simulink model "RobotX_SLAMdataCollect"  (R2014a)
settings: Solver=FixedStepDiscrete  StartTime=0.0  StopTime=inf  FixedStep=.25  RelTol=1e-3
undefined symbols (not defined in the file): Com1, Com2, Com3, Com4, DiscIntNeverNeededParam, standard
libraries: xpcseriallib x11, slrtlib x4, simulink x1, speedgoatlib x1, speedgoatlib_IO102 x1
settings Model: BufferReuse=off  Creator=wildcat  LastModifiedBy=wildcat
settings SolverCC: EnableConcurrentExecution=on
settings DataIOCC: SignalLoggingSaveFormat=ModelDataLogs
settings OptimizationCC: BlockReduction=off  OptimizeBlockIOStorage=off  BufferReuse=off  GlobalBufferReuse=off  ExpressionFolding=off  LocalBlockOutputs=off
settings DebuggingCC: UnderspecifiedInitializationDetection=Classic  StateNameClashWarn=warning
settings HardwareCC: ProdIntDivRoundTo=Zero  ProdEndianess=LittleEndian  ProdHWDeviceType=Generic->32-bit x86 compatible
settings RTWCC: SystemTargetFile=slrt.tlc  TemplateMakefile=slrt_default_tmf  Description=Simulink Real-Time  ProcessScript=slrt_make_rtw_hook  RTWCompilerOptimization=On
settings SimulinkRealTimeCC: GeneratePreprocessorConditionals=Disable all  EnableShiftOperators=on

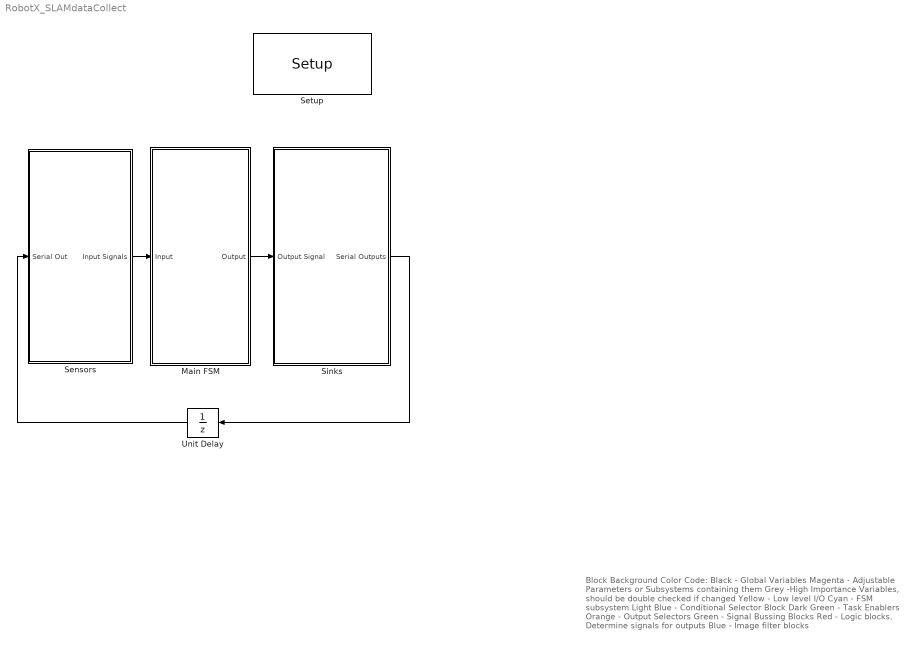
== system RobotX_SLAMdataCollect ==
  note: Block Background Color Code:
      | Black - Global Variables
      | Magenta - Adjustable Parameters or Subsystems containing them
      | Grey -High Importance Variables, should be double checked if changed
      | Yellow - Low level I/O
      | Cyan - FSM subsystem
      | Light Blue - Conditional Selector Block
      | Dark Green - Task Enablers
      | Orange - Output Selectors
      | Green - Signal Bussing Blocks
      | Red - Logic blocks. Determine signals for outputs
      | Blue - Image filter blocks
  Main FSM : Subsystem
  Sensors : Subsystem
  Setup : speedgoatlib_IO102/Setup  group=Digital output setup  id=1  range=+-5V  cal=off  pciSlot=-1  adChannelMode=Multiple-channel (enter number of channels below)  adChannel=16  adCoupling=Differential  daChannel=[1,2,3,4]  daReset=[1]  daInitValue=[0]  diChannel=[1,2,3,4,5,6,7,8]  doChannel=[1,2,3,4,5,6,7,8]  doReset=[1]  doInitValue=[0]
  Sinks : Subsystem
  Unit Delay : UnitDelay  SampleTime=-1
  wires:
  Main FSM/1(Output) -> Sinks/1(Output Signal)
  Sensors/1(Input Signals) -> Main FSM/1(Input)
  Sinks/1(Serial Outputs) -> Unit Delay/1
  Unit Delay/1 -> Sensors/1(Serial Out)

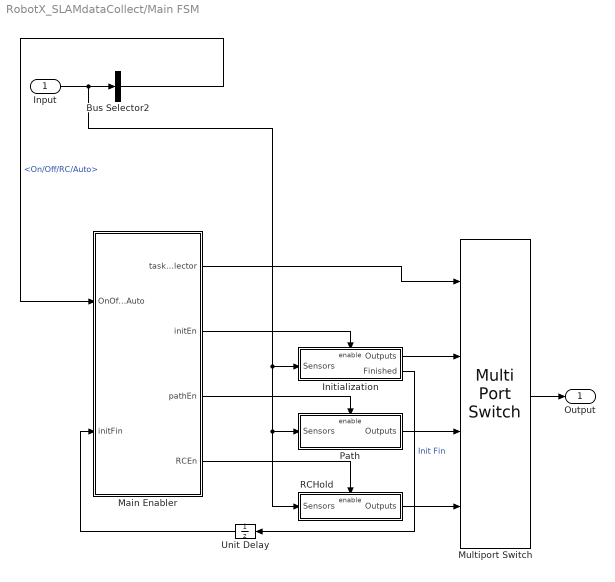
== system RobotX_SLAMdataCollect/Main FSM ==
  Input : Inport
  Bus Selector2 : BusSelector  OutputSignals=Navigation Message.On/Off/RC/Auto
  Initialization : Subsystem
  Main Enabler : MATLAB Function  TreatAsAtomicUnit=on
  Multiport Switch : MultiPortSwitch
  Path : Subsystem  TreatAsAtomicUnit=on
  RCHold : Subsystem
  Unit Delay : UnitDelay  SampleTime=-1
  Output : Outport
  wires:
  Input/1 -> Path/1(Sensors), RCHold/1(Sensors), Initialization/1(Sensors), Bus Selector2/1
  Bus Selector2/1 -> Main Enabler/1(OnOffRCAuto)  "<On/Off/RC/Auto>"
  Initialization/1(Outputs) -> Multiport Switch/2
  Path/1(Outputs) -> Multiport Switch/3
  RCHold/1(Outputs) -> Multiport Switch/4
  Main Enabler/2(initEn) -> Initialization/Enable
  Main Enabler/3(pathEn) -> Path/Enable
  Main Enabler/4(RCEn) -> RCHold/Enable
  Main Enabler/1(taskSelector) -> Multiport Switch/1
  Multiport Switch/1 -> Output/1
  Initialization/2(Finished) -> Unit Delay/1  "Init Fin"
  Unit Delay/1 -> Main Enabler/2(initFin)

== system RobotX_SLAMdataCollect/Sensors ==
  Serial Out : Inport
  Serial In : Subsystem
  Input Signals : Outport
  wires:
  Serial In/1(Serial In) -> Input Signals/1  "Sensors"
  Serial Out/1 -> Serial In/1(Serial Out)

== system RobotX_SLAMdataCollect/Sinks ==
  Output Signal : Inport
  Bus Selector : BusSelector  OutputSignals=Outputs
  data log : Subsystem  Commented=on
  Serial Outputs : Outport
  wires:
  Output Signal/1 -> Bus Selector/1
  Bus Selector/1 -> Serial Outputs/1  "<Outputs>"

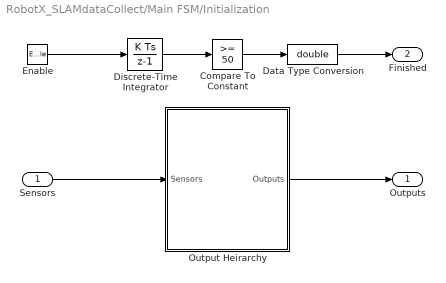
== system RobotX_SLAMdataCollect/Main FSM/Initialization ==
  Sensors : Inport
  Enable : EnablePort  ShowOutputPort=on
  Compare To Constant : simulink/Logic and Bit Operations/Compare To Constant  relop=>=  const=50  OutDataTypeStr=boolean
  Data Type Conversion : DataTypeConversion  OutDataTypeStr=double
  Discrete-Time Integrator : DiscreteIntegrator  SampleTime=-1  ICPrevOutput=DiscIntNeverNeededParam  ICPrevScaledInput=DiscIntNeverNeededParam
  Output Heirarchy : Subsystem
  Outputs : Outport
  Finished : Outport  Port=2
  wires:
  Sensors/1 -> Output Heirarchy/1(Sensors)
  Output Heirarchy/1(Outputs) -> Outputs/1
  Compare To Constant/1 -> Data Type Conversion/1
  Enable/1 -> Discrete-Time Integrator/1
  Discrete-Time Integrator/1 -> Compare To Constant/1
  Data Type Conversion/1 -> Finished/1

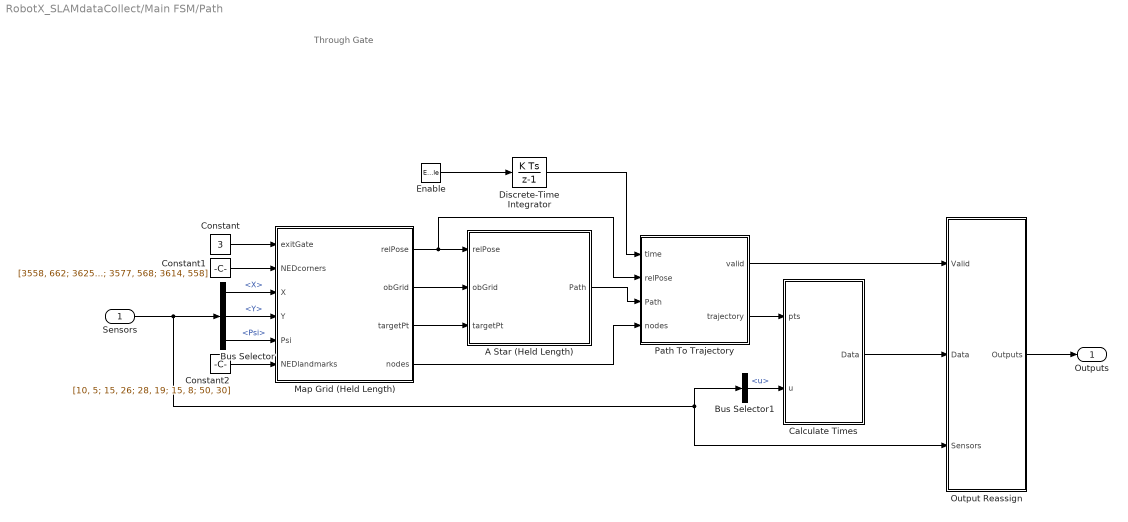
== system RobotX_SLAMdataCollect/Main FSM/Path ==
  note: Through Gate
  Sensors : Inport
  Enable : EnablePort  ShowOutputPort=on
  A Star (Held Length) : MATLAB Function  TreatAsAtomicUnit=on
  Bus Selector : BusSelector  OutputSignals=Navigation Message.Pose.X,Navigation Message.Pose.Y,Navigation Message.Pose.Psi
  Bus Selector1 : BusSelector  OutputSignals=Navigation Message.Velocity.u
  Calculate Times : MATLAB Function  TreatAsAtomicUnit=on
  Constant : Constant  Value=3
  Constant1 : Constant  Value=[3558, 662; 3625, 652; 3577, 568; 3614, 558]
  Constant2 : Constant  Value=[10, 5; 15, 26; 28, 19; 15, 8; 50, 30]
  Discrete-Time Integrator : DiscreteIntegrator  SampleTime=-1  ICPrevOutput=DiscIntNeverNeededParam  ICPrevScaledInput=DiscIntNeverNeededParam
  Map Grid (Held Length) : MATLAB Function  TreatAsAtomicUnit=on
  Output Reassign : Subsystem
  Path To Trajectory : MATLAB Function  TreatAsAtomicUnit=on
  Outputs : Outport
  wires:
  Output Reassign/1(Outputs) -> Outputs/1
  Enable/1 -> Discrete-Time Integrator/1
  Map Grid (Held Length)/1(relPose) -> A Star (Held Length)/1(relPose), Path To Trajectory/2(relPose)
  Map Grid (Held Length)/2(obGrid) -> A Star (Held Length)/2(obGrid)
  Map Grid (Held Length)/3(targetPt) -> A Star (Held Length)/3(targetPt)
  A Star (Held Length)/1(Path) -> Path To Trajectory/3(Path)
  Map Grid (Held Length)/4(nodes) -> Path To Trajectory/4(nodes)
  Constant/1 -> Map Grid (Held Length)/1(exitGate)
  Constant1/1 -> Map Grid (Held Length)/2(NEDcorners)
  Bus Selector/2 -> Map Grid (Held Length)/4(Y)  "<Y>"
  Bus Selector/3 -> Map Grid (Held Length)/5(Psi)  "<Psi>"
  Constant2/1 -> Map Grid (Held Length)/6(NEDlandmarks)
  Bus Selector/1 -> Map Grid (Held Length)/3(X)  "<X>"
  Path To Trajectory/2(trajectory) -> Calculate Times/1(pts)
  Bus Selector1/1 -> Calculate Times/2(u)  "<u>"
  Path To Trajectory/1(valid) -> Output Reassign/1("Valid ")
  Calculate Times/1(Data) -> Output Reassign/2(Data)
  Sensors/1 -> Output Reassign/3(Sensors), Bus Selector1/1, Bus Selector/1
  Discrete-Time Integrator/1 -> Path To Trajectory/1(time)

== system RobotX_SLAMdataCollect/Main FSM/RCHold ==
  Sensors : Inport
  Enable : EnablePort
  Bus Selector : BusSelector  Commented=on  OutputSignals=LCM Message.Pose.X,LCM Message.Pose.Y,LCM Message.Pose.Psi
  Output Heirarchy : Subsystem  Commented=on
  Output Heirarchy1 : Subsystem
  Set Pose : MATLAB Function  Commented=on  TreatAsAtomicUnit=on
  Outputs : Outport
  wires:
  Output Heirarchy1/1(Outputs) -> Outputs/1
  Bus Selector/1 -> Set Pose/1(X)  "<X>"
  Bus Selector/3 -> Set Pose/3(Psi)  "<Psi>"
  Bus Selector/2 -> Set Pose/2(Y)  "<Y>"
  Set Pose/1(Data) -> Output Heirarchy/1(Data)
  Sensors/1 -> Output Heirarchy1/1(Sensors), Bus Selector/1

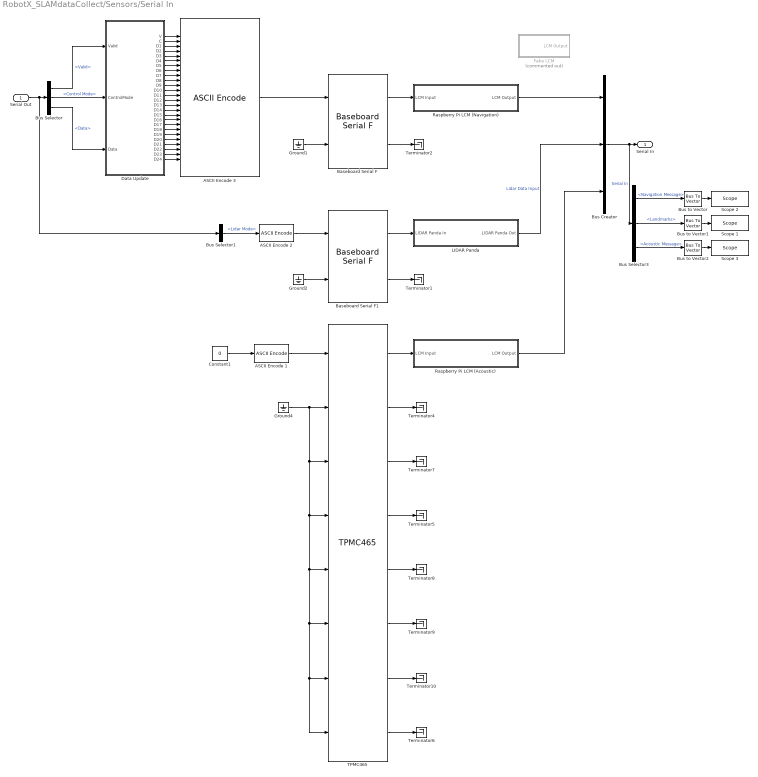
== system RobotX_SLAMdataCollect/Sensors/Serial In ==
  Serial Out : Inport
  " Raspberry Pi LCM (Acoustic)" : Subsystem
  " Raspberry Pi LCM (Navigation)" : Subsystem
  ASCII Encode 1 : xpcseriallib/ASCII Encode   format="{\"Activate\":%d} \\r\\n"  nvars=1  maxlength=20  vartypes={ 'double' }
  ASCII Encode 2 : xpcseriallib/ASCII Encode   format=SGTask:%d \r\n  nvars=1  maxlength=128  vartypes={ 'double' }
  ASCII Encode 3 : xpcseriallib/ASCII Encode   format="{\"Valid\":%d,\"Mode\":%d,\"A\":%f,\"B\":%f,\"C\":%f,\"D\":%f,\"E\":%f,\"F\":%f,\"G\":%f,\"H\":%f,\"I\":%f,\"J\":%f,\"K\":%f,\"L\":%f,\"M\":%f,\"N\":%f,\"O\":%f,\"P\":%f,\"Q\":%f,\"R\":%f,\"S\":%f,\"T\":%f,\"U\":%f,\"V\":%f,\"W\":%f,\"X\":%f} \\r\\n"  nvars=26  maxlength=450  vartypes={ 'double' }
  Baseboard Serial F : xpcseriallib/Mainboard/Baseboard Serial F  group=Basic Setup  port=1  irqnum=4  saddr1=0x3f8  saddr2=0x3e8  config=Com1/Com3  baud1=115200  parity1=Even  ndata1=7  nstop1=1  fifomode1=64 deep  rlevel1=quarter full  automode1=on  xmtfifosize1=1024  xmtdatatype1=8 bit uint null terminated  rcvfifosize1=1024  baud2=115200  parity2=Even  ndata2=7  nstop2=1  fifomode2=64 deep  rlevel2=1  automode2=on  xmtfifosize2=1024  xmtdatatype2=8 bit uint null terminated  rcvfifosize2=1024
  Baseboard Serial F1 : xpcseriallib/Mainboard/Baseboard Serial F  group=Basic Setup  port=2  irqnum=4  saddr1=0x3f8  saddr2=0x3e8  config=Com2/Com4  baud1=115200  parity1=Even  ndata1=7  nstop1=1  fifomode1=64 deep  rlevel1=quarter full  automode1=on  xmtfifosize1=1024  xmtdatatype1=8 bit uint null terminated  rcvfifosize1=1024  baud2=115200  parity2=Even  ndata2=7  nstop2=1  fifomode2=64 deep  rlevel2=quarter full  automode2=on  xmtfifosize2=1024  xmtdatatype2=8 bit uint null terminated  rcvfifosize2=1024
  Bus Creator : BusCreator  Inputs=3
  Bus Selector : BusSelector  OutputSignals=Navigation Outputs.Valid,Navigation Outputs.Control Mode,Navigation Outputs.Data
  Bus Selector1 : BusSelector  OutputSignals=Lidar Mode
  Bus Selector3 : BusSelector  OutputSignals=Navigation Message,Lidar Data Input.Landmarks,Acoustic Message
  Bus to Vector : BusToVector
  Bus to Vector1 : BusToVector
  Bus to Vector2 : BusToVector
  Constant1 : Constant  Value=0  VectorParams1D=off
  Data Update : MATLAB Function  TreatAsAtomicUnit=on
  Fake LCM : Subsystem  Commented=on
  Ground1 : Ground
  Ground2 : Ground
  Ground4 : Ground
  LIDAR Panda : Subsystem
  Scope 1 : slrtlib/Displays and Logging/Scope   scopeno=2  scopetype=File  autostart=on  viewmode=Graphical redraw  formatstr='%15.6f'  grid=on  ylimits=[0,0]  nosamples=28800  noprepostsamples=0  interleave=1  triggermode=FreeRun  triggersignal=1  trigsignalfromport=off  triggerlevel=0.0  triggerslope=Either  triggerscope=1  triggersample=0  filename=LM1_<%%%>.dat  mode=Lazy  writesize=512  autorestart=on  dynamicfilemode=on  maxwritefilesize=512*1024^2
  Scope 2 : slrtlib/Displays and Logging/Scope   scopeno=1  scopetype=File  autostart=on  viewmode=Graphical redraw  formatstr='%15.6f'  grid=on  ylimits=[0,0]  nosamples=28800  noprepostsamples=0  interleave=1  triggermode=FreeRun  triggersignal=1  trigsignalfromport=off  triggerlevel=0.0  triggerslope=Either  triggerscope=1  triggersample=0  filename=NAV1_<%%%>.dat  mode=Lazy  writesize=512  autorestart=on  dynamicfilemode=on  maxwritefilesize=512*1024^2
  Scope 3 : slrtlib/Displays and Logging/Scope   scopeno=3  scopetype=File  autostart=on  viewmode=Graphical redraw  formatstr='%15.6f'  grid=on  ylimits=[0,0]  nosamples=28800  noprepostsamples=0  interleave=1  triggermode=FreeRun  triggersignal=1  trigsignalfromport=off  triggerlevel=0.0  triggerslope=Either  triggerscope=1  triggersample=0  filename=ACO1_<%%%>.dat  mode=Lazy  writesize=512  autorestart=on  dynamicfilemode=on  maxwritefilesize=512*1024^2
  TPMC465 : speedgoatlib/IO504/TPMC465  group=Basic Setup  port=2  irqnum=9  slot=-1  transceiver1=RS232 (max 921.6kb/s)  standard1=on  baud1=115200  bauddivisor1=1  sampling1=16x (standard)  prescale1=off  parity1=Even  ndata1=7  nstop1=1  rlevel1=half full (32)  hwmode1=none  swmode1=none  xonchar1=17  xoffchar1=19  rs485auto1=off  rs485delay1=0  xmtfifosize1=1024  xmtdatatype1=8 bit uint null terminated  rcvfifosize1=1024  transceiver2=RS232 (max 921.6kb/s)  standard2=on  baud2=115200  bauddivisor2=1  sampling2=16x (standard)  prescale2=off  parity2=None  ndata2=8  nstop2=1  rlevel2=half full (32)  hwmode2=none  swmode2=none  xonchar2=17  xoffchar2=19  rs485auto2=off  rs485delay2=0  xmtfifosize2=1024  xmtdatatype2=8 bit uint null terminated  rcvfifosize2=1024  transceiver3=RS232 (max 921.6kb/s)  standard3=on  baud3=115200  bauddivisor3=1  sampling3=16x (standard)  prescale3=off  parity3=None  ndata3=8  nstop3=1  rlevel3=half full (32)  hwmode3=none  swmode3=none  xonchar3=17  xoffchar3=19  rs485auto3=off  rs485delay3=0  xmtfifosize3=1024  xmtdatatype3=8 bit uint null terminated  rcvfifosize3=1024  transceiver4=RS232 (max 921.6kb/s)  standard4=on  baud4=115200  bauddivisor4=1  sampling4=16x (standard)  prescale4=off  parity4=None  ndata4=8  nstop4=1  rlevel4=half full (32)  hwmode4=none  swmode4=none  xonchar4=17  xoffchar4=19  rs485auto4=off  rs485delay4=0  xmtfifosize4=1024  xmtdatatype4=8 bit uint null terminated  rcvfifosize4=1024  transceiver5=RS232 (max 921.6kb/s)  standard5=on  baud5=115200  bauddivisor5=1  sampling5=16x (standard)  prescale5=off  parity5=None  ndata5=8  nstop5=1  rlevel5=1  hwmode5=none  swmode5=none  xonchar5=17  xoffchar5=19  rs485auto5=off  rs485delay5=0  xmtfifosize5=1024  xmtdatatype5=8 bit uint null terminated  rcvfifosize5=1024  transceiver6=RS232 (max 921.6kb/s)  standard6=on  baud6=115200  bauddivisor6=1  sampling6=16x (standard)  prescale6=off  parity6=None  ndata6=8  nstop6=1  rlevel6=1  hwmode6=none  swmode6=none  xonchar6=17  xoffchar6=19  rs485auto6=off  rs485delay6=0  xmtfifosize6=1024  xmtdatatype6=8 bit uint null terminated  rcvfifosize6=1024  transceiver7=RS232 (max 921.6kb/s)  standard7=on  baud7=115200  bauddivisor7=1  sampling7=16x (standard)  prescale7=off  parity7=None  ndata7=8  nstop7=1  rlevel7=1  hwmode7=none  swmode7=none  xonchar7=17  xoffchar7=19  rs485auto7=off  rs485delay7=0  xmtfifosize7=1024  xmtdatatype7=8 bit uint null terminated  rcvfifosize7=1024  transceiver8=RS232 (max 921.6kb/s)  standard8=on  baud8=115200  bauddivisor8=1  sampling8=16x (standard)  prescale8=off  parity8=None  ndata8=8  nstop8=1  rlevel8=1  hwmode8=none  swmode8=none  xonchar8=17  xoffchar8=19  rs485auto8=off  rs485delay8=0  xmtfifosize8=1024  xmtdatatype8=8 bit uint null terminated  rcvfifosize8=1024
  Terminator{1..2,4..10} (9 alike) : Terminator
  Serial In : Outport
  wires:
  Baseboard Serial F1/1 -> LIDAR Panda/1(LIDAR Panda In)
  Serial Out/1 -> Bus Selector1/1, Bus Selector/1
  Baseboard Serial F/1 -> " Raspberry Pi LCM (Navigation)"/1(LCM Input)
  TPMC465/1 -> " Raspberry Pi LCM (Acoustic)"/1(LCM Input)
  ASCII Encode 3/1 -> Baseboard Serial F/1
  " Raspberry Pi LCM (Navigation)"/1(LCM Output) -> Bus Creator/1
  ASCII Encode 1/1 -> TPMC465/1
  Data Update/9(D7) -> ASCII Encode 3/9
  Data Update/11(D9) -> ASCII Encode 3/11
  Data Update/3(D1) -> ASCII Encode 3/3
  Data Update/6(D4) -> ASCII Encode 3/6
  Data Update/7(D5) -> ASCII Encode 3/7
  Data Update/2(C) -> ASCII Encode 3/2
  Data Update/5(D3) -> ASCII Encode 3/5
  Data Update/4(D2) -> ASCII Encode 3/4
  Data Update/13(D11) -> ASCII Encode 3/13
  Data Update/14(D12) -> ASCII Encode 3/14
  Data Update/1(V) -> ASCII Encode 3/1
  Data Update/12(D10) -> ASCII Encode 3/12
  Data Update/10(D8) -> ASCII Encode 3/10
  Data Update/8(D6) -> ASCII Encode 3/8
  Bus Selector/1 -> Data Update/1(Valid)  "<Valid>"
  Bus Selector/2 -> Data Update/2(ControlMode)  "<Control Mode>"
  Bus Selector/3 -> Data Update/3(Data)  "<Data>"
  Data Update/24(D22) -> ASCII Encode 3/24
  Data Update/26(D24) -> ASCII Encode 3/26
  Data Update/18(D16) -> ASCII Encode 3/18
  Data Update/23(D21) -> ASCII Encode 3/23
  Data Update/22(D20) -> ASCII Encode 3/22
  Data Update/21(D19) -> ASCII Encode 3/21
  Data Update/19(D17) -> ASCII Encode 3/19
  Data Update/17(D15) -> ASCII Encode 3/17
  Data Update/16(D14) -> ASCII Encode 3/16
  Data Update/25(D23) -> ASCII Encode 3/25
  Data Update/20(D18) -> ASCII Encode 3/20
  Data Update/15(D13) -> ASCII Encode 3/15
  " Raspberry Pi LCM (Acoustic)"/1(LCM Output) -> Bus Creator/3
  Baseboard Serial F/2 -> Terminator2/1
  Ground1/1 -> Baseboard Serial F/2
  ASCII Encode 2/1 -> Baseboard Serial F1/1
  LIDAR Panda/1(LIDAR Panda Out) -> Bus Creator/2  "Lidar Data Input"
  TPMC465/7 -> Terminator10/1
  TPMC465/5 -> Terminator8/1
  TPMC465/6 -> Terminator9/1
  TPMC465/3 -> Terminator7/1
  TPMC465/2 -> Terminator4/1
  TPMC465/4 -> Terminator5/1
  TPMC465/8 -> Terminator6/1
  Ground4/1 -> TPMC465/2, TPMC465/3, TPMC465/4, TPMC465/5, TPMC465/6, TPMC465/7, TPMC465/8
  Baseboard Serial F1/2 -> Terminator1/1
  Ground2/1 -> Baseboard Serial F1/2
  Bus Selector1/1 -> ASCII Encode 2/1  "<Lidar Mode>"
  Constant1/1 -> ASCII Encode 1/1
  Bus Creator/1 -> Bus Selector3/1, Serial In/1  "Serial In"
  Bus to Vector/1 -> Scope 2/1
  Bus Selector3/1 -> Bus to Vector/1  "<Navigation Message>"
  Bus to Vector1/1 -> Scope 1/1
  Bus Selector3/2 -> Bus to Vector1/1  "<Landmarks>"
  Bus to Vector2/1 -> Scope 3/1
  Bus Selector3/3 -> Bus to Vector2/1  "<Acoustic Message>"

== system RobotX_SLAMdataCollect/Sinks/data log ==
  note: need to play with the boat to figure out how this works properly
  Output signal : Inport
  "Scope " : slrtlib/Displays and Logging/Scope   scopeno=1  scopetype=File  autostart=on  viewmode=Graphical redraw  formatstr='%15.6f'  grid=on  ylimits=[0,0]  nosamples=250  noprepostsamples=0  interleave=1  triggermode=Signal triggering  triggersignal=1  trigsignalfromport=on  triggerlevel=1  triggerslope=Rising  triggerscope=1  triggersample=0  filename=data.dat  mode=Lazy  writesize=512  autorestart=off  dynamicfilemode=off  maxwritefilesize=512*1024^2
  wires:
  Output signal/1 -> ?

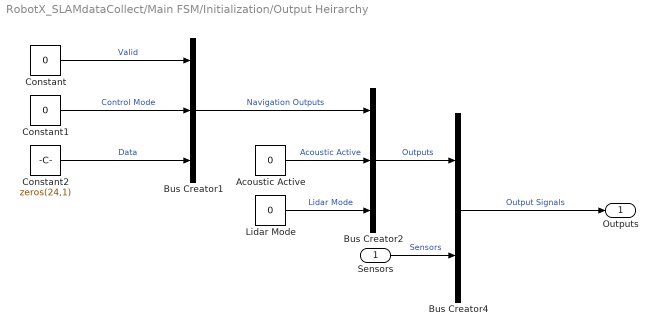
== system RobotX_SLAMdataCollect/Main FSM/Initialization/Output Heirarchy ==
  Sensors : Inport
  Acoustic Active : Constant  Value=0
  Bus Creator1 : BusCreator  Inputs=3
  Bus Creator2 : BusCreator  Inputs=3
  Bus Creator4 : BusCreator  Inputs=2
  Constant : Constant  Value=0
  Constant1 : Constant  Value=0
  Constant2 : Constant  Value=zeros(24,1)
  Lidar Mode : Constant  Value=0
  Outputs : Outport
  wires:
  Sensors/1 -> Bus Creator4/2  "Sensors"
  Bus Creator4/1 -> Outputs/1  "Output Signals"
  Constant/1 -> Bus Creator1/1  "Valid"
  Constant1/1 -> Bus Creator1/2  "Control Mode"
  Constant2/1 -> Bus Creator1/3  "Data"
  Bus Creator1/1 -> Bus Creator2/1  "Navigation Outputs"
  Acoustic Active/1 -> Bus Creator2/2  "Acoustic Active"
  Lidar Mode/1 -> Bus Creator2/3  "Lidar Mode"
  Bus Creator2/1 -> Bus Creator4/1  "Outputs"

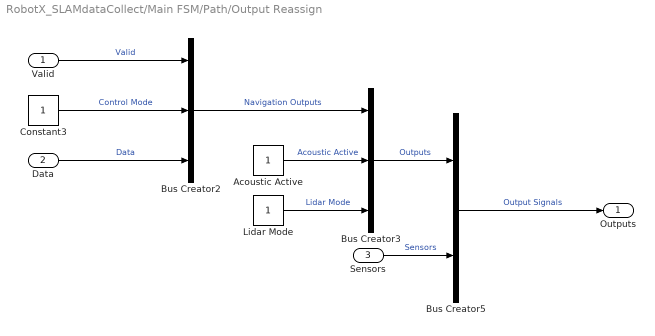
== system RobotX_SLAMdataCollect/Main FSM/Path/Output Reassign ==
  "Valid " : Inport
  Data : Inport  Port=2
  Sensors : Inport  Port=3
  Acoustic Active : Constant
  Bus Creator2 : BusCreator  Inputs=3
  Bus Creator3 : BusCreator  Inputs=3
  Bus Creator5 : BusCreator  Inputs=2
  Constant3 : Constant
  Lidar Mode : Constant
  Outputs : Outport
  wires:
  Sensors/1 -> Bus Creator5/2  "Sensors"
  Bus Creator5/1 -> Outputs/1  "Output Signals"
  "Valid "/1 -> Bus Creator2/1  "Valid"
  Constant3/1 -> Bus Creator2/2  "Control Mode"
  Data/1 -> Bus Creator2/3  "Data"
  Bus Creator2/1 -> Bus Creator3/1  "Navigation Outputs"
  Acoustic Active/1 -> Bus Creator3/2  "Acoustic Active"
  Lidar Mode/1 -> Bus Creator3/3  "Lidar Mode"
  Bus Creator3/1 -> Bus Creator5/1  "Outputs"

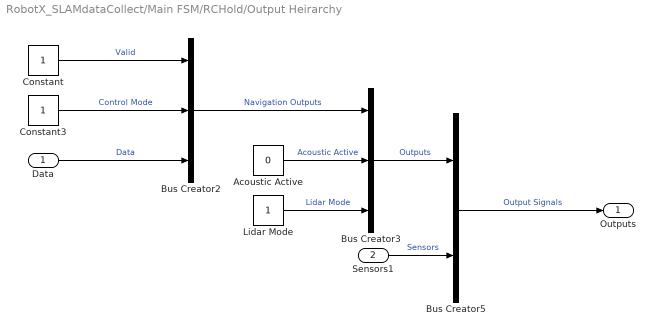
== system RobotX_SLAMdataCollect/Main FSM/RCHold/Output Heirarchy ==
  Data : Inport
  Sensors1 : Inport  Port=2
  Acoustic Active : Constant  Value=0
  Bus Creator2 : BusCreator  Inputs=3
  Bus Creator3 : BusCreator  Inputs=3
  Bus Creator5 : BusCreator  Inputs=2
  Constant : Constant
  Constant3 : Constant
  Lidar Mode : Constant
  Outputs : Outport
  wires:
  Sensors1/1 -> Bus Creator5/2  "Sensors"
  Bus Creator5/1 -> Outputs/1  "Output Signals"
  Constant/1 -> Bus Creator2/1  "Valid"
  Constant3/1 -> Bus Creator2/2  "Control Mode"
  Data/1 -> Bus Creator2/3  "Data"
  Bus Creator2/1 -> Bus Creator3/1  "Navigation Outputs"
  Acoustic Active/1 -> Bus Creator3/2  "Acoustic Active"
  Lidar Mode/1 -> Bus Creator3/3  "Lidar Mode"
  Bus Creator3/1 -> Bus Creator5/1  "Outputs"

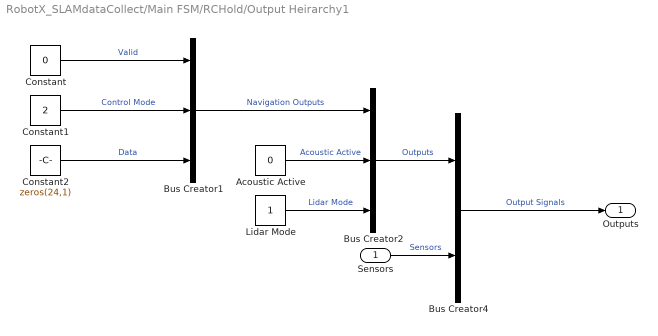
== system RobotX_SLAMdataCollect/Main FSM/RCHold/Output Heirarchy1 ==
  Sensors : Inport
  Acoustic Active : Constant  Value=0
  Bus Creator1 : BusCreator  Inputs=3
  Bus Creator2 : BusCreator  Inputs=3
  Bus Creator4 : BusCreator  Inputs=2
  Constant : Constant  Value=0
  Constant1 : Constant  Value=2
  Constant2 : Constant  Value=zeros(24,1)
  Lidar Mode : Constant
  Outputs : Outport
  wires:
  Sensors/1 -> Bus Creator4/2  "Sensors"
  Bus Creator4/1 -> Outputs/1  "Output Signals"
  Constant/1 -> Bus Creator1/1  "Valid"
  Constant1/1 -> Bus Creator1/2  "Control Mode"
  Constant2/1 -> Bus Creator1/3  "Data"
  Bus Creator1/1 -> Bus Creator2/1  "Navigation Outputs"
  Acoustic Active/1 -> Bus Creator2/2  "Acoustic Active"
  Lidar Mode/1 -> Bus Creator2/3  "Lidar Mode"
  Bus Creator2/1 -> Bus Creator4/1  "Outputs"

== system RobotX_SLAMdataCollect/Sensors/Serial In/ Raspberry Pi LCM (Acoustic) ==
  LCM Input : Inport
  ASCII Decode 6 : xpcseriallib/ASCII Decode   format=Deploy:%1u, Elapsed:%g, Bearing1:%g Bearing2:%g \r\n  nvars=4  vartypes={}
  Bus Creator : BusCreator  Inputs=2
  Bus Creator1 : BusCreator  Inputs=3
  FIFO ASCII read 1 : xpcseriallib/FIFO ASCII read   header={'Deploy:'}  term=[13 10]  hold=Zero output if no new data  enable=off  maxsize=1024  outputtype=8 bit uint null terminated  sampletime=-1
  LCM Output : Outport
  wires:
  LCM Input/1 -> FIFO ASCII read 1/1
  FIFO ASCII read 1/1 -> ASCII Decode 6/1
  ASCII Decode 6/3 -> Bus Creator/1  "Horizontal Bearing"
  ASCII Decode 6/4 -> Bus Creator/2  "Vertical Bearing"
  Bus Creator/1 -> Bus Creator1/3  "Bearings"
  ASCII Decode 6/2 -> Bus Creator1/2  "Elapsed Time"
  ASCII Decode 6/1 -> Bus Creator1/1  "Deployed"
  Bus Creator1/1 -> LCM Output/1  "Acoustic Message"

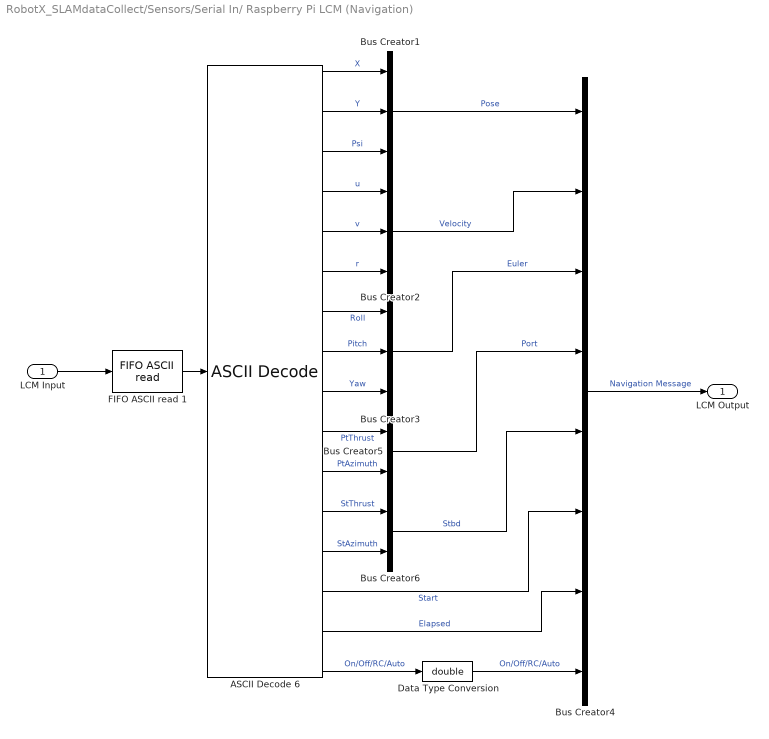
== system RobotX_SLAMdataCollect/Sensors/Serial In/ Raspberry Pi LCM (Navigation) ==
  LCM Input : Inport
  ASCII Decode 6 : xpcseriallib/ASCII Decode   format=P1:%f P2:%f P3:%f V1:%f V2:%f V3:%f E1:%f E2:%f E3:%f Pt1:%f Pt2:%f St1:%f St2:%f Start:%f Elapsed:%f RC:%d \r\n  nvars=16  vartypes={}
  Bus Creator1 : BusCreator  Inputs=3
  Bus Creator2 : BusCreator  Inputs=3
  Bus Creator3 : BusCreator  Inputs=3
  Bus Creator4 : BusCreator  Inputs=8
  Bus Creator5 : BusCreator  Inputs=2
  Bus Creator6 : BusCreator  Inputs=2
  Data Type Conversion : DataTypeConversion  OutDataTypeStr=double
  FIFO ASCII read 1 : xpcseriallib/FIFO ASCII read   header={'P1:'}  term=[13 10]  hold=Zero output if no new data  enable=off  maxsize=1024  outputtype=8 bit uint null terminated  sampletime=-1
  LCM Output : Outport
  wires:
  LCM Input/1 -> FIFO ASCII read 1/1
  FIFO ASCII read 1/1 -> ASCII Decode 6/1
  Bus Creator4/1 -> LCM Output/1  "Navigation Message"
  ASCII Decode 6/1 -> Bus Creator1/1  "X"
  ASCII Decode 6/2 -> Bus Creator1/2  "Y"
  ASCII Decode 6/3 -> Bus Creator1/3  "Psi"
  Bus Creator1/1 -> Bus Creator4/1  "Pose"
  ASCII Decode 6/4 -> Bus Creator2/1  "u"
  ASCII Decode 6/5 -> Bus Creator2/2  "v"
  Bus Creator2/1 -> Bus Creator4/2  "Velocity"
  ASCII Decode 6/7 -> Bus Creator3/1  "Roll"
  ASCII Decode 6/8 -> Bus Creator3/2  "Pitch"
  ASCII Decode 6/9 -> Bus Creator3/3  "Yaw"
  Bus Creator3/1 -> Bus Creator4/3  "Euler"
  Bus Creator5/1 -> Bus Creator4/4  "Port"
  Bus Creator6/1 -> Bus Creator4/5  "Stbd"
  ASCII Decode 6/12 -> Bus Creator6/1  "StThrust"
  ASCII Decode 6/13 -> Bus Creator6/2  "StAzimuth"
  ASCII Decode 6/10 -> Bus Creator5/1  "PtThrust"
  ASCII Decode 6/11 -> Bus Creator5/2  "PtAzimuth"
  ASCII Decode 6/14 -> Bus Creator4/6  "Start"
  ASCII Decode 6/15 -> Bus Creator4/7  "Elapsed"
  ASCII Decode 6/16 -> Data Type Conversion/1  "On/Off/RC/Auto"
  Data Type Conversion/1 -> Bus Creator4/8  "On/Off/RC/Auto"
  ASCII Decode 6/6 -> Bus Creator2/3  "r"

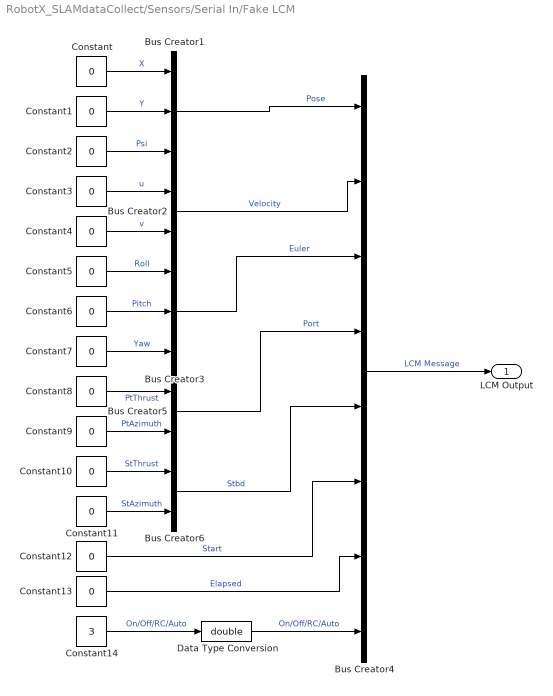
== system RobotX_SLAMdataCollect/Sensors/Serial In/Fake LCM ==
  Bus Creator1 : BusCreator  Inputs=3
  Bus Creator2 : BusCreator  Inputs=2
  Bus Creator3 : BusCreator  Inputs=3
  Bus Creator4 : BusCreator  Inputs=8
  Bus Creator5 : BusCreator  Inputs=2
  Bus Creator6 : BusCreator  Inputs=2
  Constant{,1..13} (14 alike) : Constant  Value=0
  Constant14 : Constant  Value=3
  Data Type Conversion : DataTypeConversion  OutDataTypeStr=double
  LCM Output : Outport
  wires:
  Bus Creator4/1 -> LCM Output/1  "LCM Message"
  Constant/1 -> Bus Creator1/1  "X"
  Constant1/1 -> Bus Creator1/2  "Y"
  Constant2/1 -> Bus Creator1/3  "Psi"
  Bus Creator1/1 -> Bus Creator4/1  "Pose"
  Constant3/1 -> Bus Creator2/1  "u"
  Constant4/1 -> Bus Creator2/2  "v"
  Bus Creator2/1 -> Bus Creator4/2  "Velocity"
  Constant5/1 -> Bus Creator3/1  "Roll"
  Constant6/1 -> Bus Creator3/2  "Pitch"
  Constant7/1 -> Bus Creator3/3  "Yaw"
  Bus Creator3/1 -> Bus Creator4/3  "Euler"
  Bus Creator5/1 -> Bus Creator4/4  "Port"
  Bus Creator6/1 -> Bus Creator4/5  "Stbd"
  Constant10/1 -> Bus Creator6/1  "StThrust"
  Constant11/1 -> Bus Creator6/2  "StAzimuth"
  Constant8/1 -> Bus Creator5/1  "PtThrust"
  Constant9/1 -> Bus Creator5/2  "PtAzimuth"
  Constant12/1 -> Bus Creator4/6  "Start"
  Constant13/1 -> Bus Creator4/7  "Elapsed"
  Constant14/1 -> Data Type Conversion/1  "On/Off/RC/Auto"
  Data Type Conversion/1 -> Bus Creator4/8  "On/Off/RC/Auto"

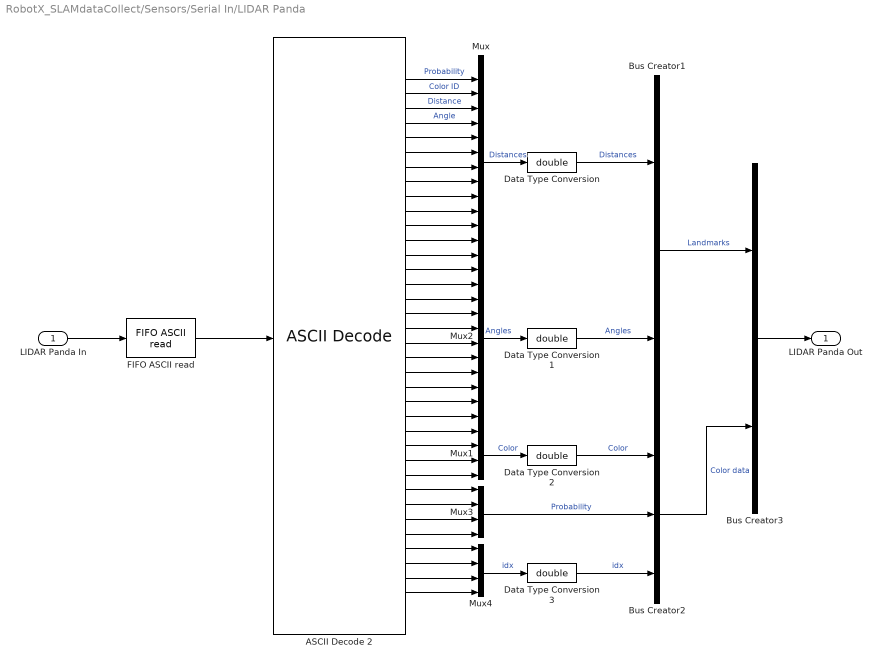
== system RobotX_SLAMdataCollect/Sensors/Serial In/LIDAR Panda ==
  LIDAR Panda In : Inport
  ASCII Decode 2 : xpcseriallib/ASCII Decode   format=A:%d B:%d C:%d E:%d F:%d G:%d H:%d I:%d J:%d K:%d L:%d M:%d N:%d O:%d P:%d Q:%d R:%d S:%d T:%d U:%d V:%d W:%d X:%d C1:%d C2:%d C3:%d C4:%d P1:%f P2:%f P3:%f P4:%f I1:%d I2:%d I3:%d I4:%d \r\n  nvars=36  vartypes={}
  Bus Creator1 : BusCreator  Inputs=2
  Bus Creator2 : BusCreator  Inputs=3
  Bus Creator3 : BusCreator  Inputs=2
  Data Type Conversion{,1..3} (4 alike) : DataTypeConversion  OutDataTypeStr=double
  "FIFO ASCII read " : xpcseriallib/FIFO ASCII read   header={'A:'}  term=[13 10]  hold=Zero output if no new data  enable=off  maxsize=1024  outputtype=8 bit uint null terminated  sampletime=-1
  Mux : Mux  Inputs=12
  Mux1 : Mux
  Mux2 : Mux  Inputs=12
  Mux3 : Mux
  Mux4 : Mux
  LIDAR Panda Out : Outport
  wires:
  LIDAR Panda In/1 -> "FIFO ASCII read "/1
  "FIFO ASCII read "/1 -> ASCII Decode 2/1
  ASCII Decode 2/3 -> Mux/3  "Distance"
  ASCII Decode 2/2 -> Mux/2  "Color ID"
  ASCII Decode 2/4 -> Mux/4  "Angle"
  ASCII Decode 2/1 -> Mux/1  "Probability"
  ASCII Decode 2/7 -> Mux/7
  ASCII Decode 2/10 -> Mux/10
  ASCII Decode 2/11 -> Mux/11
  ASCII Decode 2/6 -> Mux/6
  ASCII Decode 2/8 -> Mux/8
  ASCII Decode 2/9 -> Mux/9
  ASCII Decode 2/12 -> Mux/12
  ASCII Decode 2/5 -> Mux/5
  ASCII Decode 2/13 -> Mux2/1
  ASCII Decode 2/15 -> Mux2/3
  ASCII Decode 2/22 -> Mux2/10
  ASCII Decode 2/23 -> Mux2/11
  ASCII Decode 2/17 -> Mux2/5
  ASCII Decode 2/18 -> Mux2/6
  ASCII Decode 2/14 -> Mux2/2
  ASCII Decode 2/24 -> Mux2/12
  ASCII Decode 2/20 -> Mux2/8
  ASCII Decode 2/19 -> Mux2/7
  ASCII Decode 2/21 -> Mux2/9
  ASCII Decode 2/16 -> Mux2/4
  ASCII Decode 2/25 -> Mux1/1
  ASCII Decode 2/28 -> Mux1/4
  ASCII Decode 2/26 -> Mux1/2
  ASCII Decode 2/27 -> Mux1/3
  ASCII Decode 2/30 -> Mux3/2
  ASCII Decode 2/31 -> Mux3/3
  ASCII Decode 2/32 -> Mux3/4
  ASCII Decode 2/29 -> Mux3/1
  ASCII Decode 2/36 -> Mux4/4
  ASCII Decode 2/34 -> Mux4/2
  ASCII Decode 2/35 -> Mux4/3
  ASCII Decode 2/33 -> Mux4/1
  Mux/1 -> Data Type Conversion/1  "Distances"
  Mux2/1 -> Data Type Conversion1/1  "Angles"
  Mux1/1 -> Data Type Conversion2/1  "Color"
  Mux3/1 -> Bus Creator2/2  "Probability"
  Mux4/1 -> Data Type Conversion3/1  "idx"
  Bus Creator1/1 -> Bus Creator3/1  "Landmarks"
  Bus Creator2/1 -> Bus Creator3/2  "Color data"
  Bus Creator3/1 -> LIDAR Panda Out/1
  Data Type Conversion/1 -> Bus Creator1/1  "Distances"
  Data Type Conversion1/1 -> Bus Creator1/2  "Angles"
  Data Type Conversion2/1 -> Bus Creator2/1  "Color"
  Data Type Conversion3/1 -> Bus Creator2/3  "idx"

== matlab function RobotX_SLAMdataCollect/Main FSM/Main Enabler ==
  data: taskSelector output; initEn output; pathEn output; RCEn output; OnOffRCAuto input; initFin input
function [taskSelector,initEn,pathEn,RCEn] = taskEnabler(OnOffRCAuto, initFin)
%Written by Anderson Lebbad on July 19, 2013
%Last Edited: Edward Zhu on June 2, 2014
%   Substring search for task was written in
%   Case switches were redundant, combined with first set of if statements

%Changes the value of MainMode and the enablers for the tasks within the
%Main FSM.

% Initialize enable signals
RCEn = 0;
initEn = 0;
pathEn = 0;

% Set enable signals based on state completion
if initFin == 0
    initEn = 1;
    taskSelector = 1;
elseif OnOffRCAuto ~= 3
    RCEn = 1;
    taskSelector = 3;
else
    pathEn = 1;
    taskSelector = 2;
end

== matlab function RobotX_SLAMdataCollect/Main FSM/Path/Calculate Times ==
  data: pts input; u input; Data output
function Data = calcTimes(pts, u)
%Written by Anderson Lebbad on August 9, 2014
%Last Edited:

%Calculates times for the boat to get to points for a trajectory, and
%formats Data for communication

%Initialize
Data = zeros(24,1);
traj = zeros(8,3);
traj(:,1:2) = pts;



for k = 2:8
    %Calculate distance to travel from last point
    distTravel = sqrt(sum((pts(k-1,:)-pts(k,:)).^2));
    %Assume 1m per second speed
    traj(k,3) = traj(k-1,3) + distTravel;
    %Add time based off initial velocity to get to first point past initial
    if k == 2
        traj(k,3) = traj(k,3) + 2.5*abs(2-u);
    end
end


%Output Data
for i=1:8
    for j = 1:3
        Data(3*(i-1)+j) = traj(i,j);
    end
end

== matlab function RobotX_SLAMdataCollect/Sensors/Serial In/Data Update ==
  data: Valid input; ControlMode input; V output; C output; Data input; D1 output; D2 output; D3 output; D4 output; D5 output; D6 output; D7 output; D8 output; D9 output; D10 output; D11 output; D12 output; D13 output; D14 output; D15 output; D16 output; D17 output; D18 output; D19 output; D20 output; D21 output; D22 output; D23 output; D24 output
function [V,C,D1,D2,D3,D4,D5,D6,D7,D8,D9,D10,D11,D12,D13,D14,D15,D16,D17,...
    D18,D19,D20,D21,D22,D23,D24] = dataSplit(Valid,ControlMode,Data)
%Written by Anderson Lebbad on August 10, 2014
%Last Edited by: Anderson Lebbad on September 11, 2014

%This function splits the data vector into the twelve channels it is
%composed of for communication

persistent HoldData

if isempty(HoldData)
    HoldData = zeros(26,1);
end

if Valid == 1
    HoldData(1) = Valid;
    HoldData(2) = ControlMode;
    HoldData(3) = Data(1);
    HoldData(4) = Data(2);
    HoldData(5) = Data(3);
    HoldData(6) = Data(4);
    HoldData(7) = Data(5);
    HoldData(8) = Data(6);
    HoldData(9) = Data(7);
    HoldData(10) = Data(8);
    HoldData(11) = Data(9);
    HoldData(12) = Data(10);
    HoldData(13) = Data(11);
    HoldData(14) = Data(12);
    HoldData(15) = Data(13);
    HoldData(16) = Data(14);
    HoldData(17) = Data(15);
    HoldData(18) = Data(16);
    HoldData(19) = Data(17);
    HoldData(20) = Data(18);
    HoldData(21) = Data(19);
    HoldData(22) = Data(20);
    HoldData(23) = Data(21);
    HoldData(24) = Data(22);
    HoldData(25) = Data(23);
    HoldData(26) = Data(24);
end

V = HoldData(1);
C = HoldData(2);
D1 = HoldData(3);
D2 = HoldData(4);
D3 = HoldData(5);
D4 = HoldData(6);
D5 = HoldData(7);
D6 = HoldData(8);
D7 = HoldData(9);
D8 = HoldData(10);
D9 = HoldData(11);
D10 = HoldData(12);
D11 = HoldData(13);
D12 = HoldData(14);
D13 = HoldData(15);
D14 = HoldData(16);
D15 = HoldData(17);
D16 = HoldData(18);
D17 = HoldData(19);
D18 = HoldData(20);
D19 = HoldData(21);
D20 = HoldData(22);
D21 = HoldData(23);
D22 = HoldData(24);
D23 = HoldData(25);
D24 = HoldData(26);

end

== matlab function RobotX_SLAMdataCollect/Main FSM/RCHold/Set Pose ==
  data: X input; Data output; Y input; Psi input
function Data = setPose(X,Y,Psi)
%Written by Anderson Lebbad on August 9, 2014
%Last Edited:

%This function passes the current pose data with a heading offset as the
%desired pose for the station keeping controller to use.

persistent holdPose

if isempty(holdPose)
    holdPose = [X Y Psi];
end

%Initialize Data variable
Data = zeros(12,1);

%Set desired pose
Data(1) = holdPose(1);
Data(2) = holdPose(2);
Data(3) = holdPose(3);

== matlab function RobotX_SLAMdataCollect/Main FSM/Path/A Star (Held Length) ==
  data: relPose input; Path output; obGrid input; targetPt input
function Path  = AStarHeldLengthDebug( relPose, obGrid, targetPt )
%Written By Anderson Lebbad on August 27, 2014
%Last Edited on:

%This funtion executes an A* method for path planning given the current
%position of the vessel, the target position for the vessel to reach, and
%a map of obstacles to avoid. The A* method is well documented here:
% www.policyalmanac.org/games/aStarTutorial.htm

%% Define list sizes
[m,n] = size(obGrid);
gridPts = m*n;

%Initialize a path output variable
Path = nan(gridPts,2);
%Initialize variable to track if a solution has been found
solution_found = 0;

%Track the XY coordinates of each point to be evaluated
open_list_XY = nan(gridPts,2);
%Track the calculated F, G, and H weights (where G is the movement cost to
%get to the point, H is the Hypothetical cost to reach the target from that
%point before the full path is evaluated, and F is the sum of both G and H
%costs) for the points being evaluated
open_list_FGH = nan(gridPts,3);
%Track the coordinates of the parent for each of the points being evaluated
open_list_parent = nan(gridPts,2);

%Track the XY coordinates of each point that has been fully evaluated
closed_list_XY = nan(gridPts,2);
%Track the parent coordinate of each point that has been fully evaluated
closed_list_parent = nan(gridPts,2);
emptyClosed = find(isnan(closed_list_XY(:,1)));

%Relative indices to neighboring points of the square, to be used for
%evaluating potential candidates for the open list
neighbors_XY = [-1,-1;-1,0;-1,1;0,1;1,1;1,0;1,-1;0,-1];
neighbors_G = [14;10;14;10;14;10;14;10];

%Make the current pose (in the relative coordinates of the field) the first
%point in the open list
open_list_XY(1,:) = relPose;
current_XY = relPose;
%Set movement cost of this point to zero
open_list_FGH(1,2) = 0;
%Calculate hypothetical cost
open_list_FGH(1,3) = 10*(abs(targetPt(1)-relPose(1))+abs(targetPt(2)-relPose(2)));
%Sum is full cost
open_list_FGH(1,1) = open_list_FGH(1,2) + open_list_FGH(1,3);

%Create a list of invalid pts
%obstacles are invalid
[row, col] = find(obGrid == -1);
%outside the edges are invalid
left = [0:m+1;zeros(1,m+2)]';
right = [0:m+1;(n+1)*ones(1,m+2)]';
bottom = [zeros(1,n);1:n]';
top = [(m+1)*ones(1,n);1:n]';
invalid_pts = [row,col;left;right;bottom;top];
invalid_pts = sortrows(invalid_pts);
%Loop while there are points on the open list
while sum(~isnan(open_list_XY(:,1))) >= 1
    %% Current Square
    
    %Find the lowest F cost square on the open list, checking newer entries
    %over older. This is done by flipping the list up/down to get newer
    %entries to evaluate first. This is marked as the current square
    [~,idxI] = min(flipud(open_list_FGH(:,1)));
    CurrentSquare = gridPts - idxI(1) + 1;
    current_XY = open_list_XY(CurrentSquare,:);
    current_G = open_list_FGH(CurrentSquare,2);
    
    %Find the first empty element in the closed list, and replace the place
    %holder with the information for the current square
    emptyClosed = find(isnan(closed_list_XY(:,1)));
    closed_list_XY(emptyClosed(1),:) = current_XY;
    closed_list_parent(emptyClosed(1),:) = open_list_parent(CurrentSquare,:);
    %Remove the current square from the open list now that it is on the
    %closed list
    open_list_XY(CurrentSquare,:) = NaN;
    open_list_FGH(CurrentSquare,:) = NaN;
    open_list_parent(CurrentSquare,:) = NaN;
    
    %If the current point that just got added to the closed list is the
    %target point, exit the loop because a complete path can be traced
    if (current_XY(1) == targetPt(1)) && (current_XY(2) == targetPt(2))
        solution_found = 1;
        break
    end
    
    %% Check adjacent squares
    
    %Create a list of points around the current point and check their G
    %value
    rel_list_XY = [neighbors_XY(:,1)+current_XY(1) neighbors_XY(:,2)+current_XY(2)];
    rel_list_G = neighbors_G + current_G;
    rel_list_H = 10*(abs(targetPt(1)-rel_list_XY(:,1))+abs(targetPt(2)-rel_list_XY(:,2)));
    rel_list_F = rel_list_G + rel_list_H;
    
    %% Check walkable / on closed list
    
    %Order closed list for finding relative list points on it
    closed_list_XY_sorted = sortrows(closed_list_XY);
    %Mark members of relative list if on closed list
    on_closed = ismember(rel_list_XY,closed_list_XY_sorted,'rows');
    rel_list_XY(on_closed,:) = NaN;
    rel_list_F(on_closed) = NaN;
    rel_list_G(on_closed) = NaN;
    rel_list_H(on_closed) = NaN;
    %Check to see if members of relative list are either obstacles or out
    %of bounds
    invalid = ismember(rel_list_XY,invalid_pts,'rows');
    rel_list_XY(invalid,:) = NaN;
    rel_list_F(invalid) = NaN;
    rel_list_G(invalid) = NaN;
    rel_list_H(invalid) = NaN;
    valid = ~isnan(rel_list_XY(:,1));
    validIdx = find(valid);
    
    %% Calculate F and H, and add penalty weights to G scores
    
    if ~isempty(rel_list_XY)
        rel_list_G(valid) = rel_list_G(valid) + 20.*obGrid(rel_list_XY(valid,1)+m*(rel_list_XY(valid,2)-1));
        rel_list_F(valid) = rel_list_G(valid) + rel_list_H(valid);
        
        %% Check if on open list, if not add to it
        
        %Order open list for finding relative list points on it
        [open_list_XY_sorted, idx] = sortrows(open_list_XY);
        %Check to see if relative list points are on open list
        [rel_on_open, open_on_rel_list] = ismember(rel_list_XY(valid,:),open_list_XY_sorted,'rows');
        rel_not_on_open = validIdx(~rel_on_open);
        rel_on_open = validIdx(rel_on_open);
        %Only care about indices that are actually found, remove the ones that
        %aren't
        open_on_rel = idx(open_on_rel_list(open_on_rel_list ~= 0));
        %Whichever points that are not on the open list are
        %added to the open list (in the first available empty slots)
        num_not_on_open = length(rel_not_on_open);
        num_on_open = length(rel_on_open);
        emptyOpen = find(isnan(open_list_XY(:,1)));
        if num_not_on_open >= 1
            open_list_XY(emptyOpen(1:num_not_on_open),:) = rel_list_XY(rel_not_on_open,:);
            open_list_FGH(emptyOpen(1:num_not_on_open),:) = ...
                [rel_list_F(rel_not_on_open) rel_list_G(rel_not_on_open) rel_list_H(rel_not_on_open)];
            open_list_parent(emptyOpen(1:num_not_on_open),1) = current_XY(1);
            open_list_parent(emptyOpen(1:num_not_on_open),2) = current_XY(2);
            %Remove members of the relative list that were just put on the open
            %list (only care about the F and G, the XY and H are not updated past
            %this point)
            rel_list_F(~rel_on_open) = NaN;
            rel_list_G(~rel_on_open) = NaN;
        end
        
        %% Check G cost of rest to see if it should be updated
        
        if num_on_open >= 1
            %Find the G values of the points that are on the open list and compare
            %them to the G values for the same points on the relative list. Track
            %which G values are lower on the relative list
            lower_G_list = rel_list_G(rel_on_open) < open_list_FGH(open_on_rel,2);
            rel_idx = find(rel_on_open);
            lower_G = rel_idx(lower_G_list);
            %Replace the G and F values with the new lower ones, and update parent
            open_list_FGH(open_on_rel(lower_G_list),1:2) = [rel_list_F(lower_G) rel_list_G(lower_G)];
            open_list_parent(open_on_rel(lower_G_list),1) = current_XY(1);
            open_list_parent(open_on_rel(lower_G_list),2) = current_XY(2);
        end
        
    end
    
    %% Organize list for searching
    
    %Negates the F and H cost for to be able to descending rowsort, then negates
    %back to original values
    open_list_FGH = -open_list_FGH;
    [open_list_FGH,idx] = sortrows(open_list_FGH,[1 3]); %Sort focusing on F first, then H
    open_list_FGH = -open_list_FGH;
    open_list_XY = open_list_XY(idx,:);
    open_list_parent = open_list_parent(idx,:);
    
end

%% If solution is found, generate path

%Generate path by recursively checking parent values
if solution_found
    %Create a list of the path points, for organizational purposes for
    %outputting later
    PathList = Path;
    %Set first element as current position (the goal point)
    PathList(1,:) = current_XY;
    %Track current square's location on closed list
    CurrentSquareClosed = emptyClosed(1);
    %Create an incrementing variable for path elements
    next_index = 2;
    %Loop until there is no parent square (start square)
    while ~isnan(closed_list_parent(CurrentSquareClosed))
        %Next path element is the current element's parent
        PathList(next_index,:) = closed_list_parent(CurrentSquareClosed,:);
        %Order closed list for finding parents on it
        [closed_list_XY_sorted, idx] = sortrows(closed_list_XY);
        %Find the next element and make it the current element
        [~,locs] = ismember(closed_list_parent(CurrentSquareClosed,:),closed_list_XY_sorted,'rows');
        CurrentSquareClosed = idx(locs(1));
        %Increment the next index
        next_index = next_index + 1;
    end
    %Get the length of the path
    PathLength = next_index-1;
    %Path list is from finish to start, so flip and output
    Path(1:PathLength,:) = PathList(PathLength:-1:1,:);
end

end

== matlab function RobotX_SLAMdataCollect/Main FSM/Path/Map Grid (Held Length) ==
  data: exitGate input; relPose output; NEDcorners input; X input; Y input; Psi input; NEDlandmarks input; obGrid output; targetPt output; nodes output
function [relPose,obGrid,targetPt,nodes] = MapGridHeldLength(exitGate,NEDcorners,X,Y,Psi,NEDlandmarks)
%Written By Anderson Lebbad on September 3, 2014
%Last Edited on:

%This function takes in the exit gate identifier, the converted coordinates
%(from GPS to NED) of the bounding box of the OD/OA task, the current pose
%and the landmark list from SLAM - and generates a grid, as well as
%relative location of the vessel and the exit gate in that grid for the A*
%planner. This grid is a fixed size, so the relative size of each region
%can vary slightly depending upon the size of the bounded region sent to
%it.

%% Create node map (conversion between grid coordinates and NED coordinates)

cells_vert = 25;
cells_horiz = 10;

%Create edge devisions - corners must be ordered. First row is the bottom
%left coordinate, then bottom right is second, followed by top left,
%and finally top right. Only need top and bottom, will segment vertically
%in loop
top_edge = (0:cells_horiz-1)'*...
    [(NEDcorners(4,1)-NEDcorners(3,1))/(cells_horiz-1) (NEDcorners(4,2)-NEDcorners(3,2))/(cells_horiz-1)]+...
    ones(cells_horiz,1)*NEDcorners(3,:);
bottom_edge = (0:1:cells_horiz-1)'*...
    [(NEDcorners(2,1)-NEDcorners(1,1))/(cells_horiz-1) (NEDcorners(2,2)-NEDcorners(1,2))/(cells_horiz-1)]+...
    ones(cells_horiz,1)*NEDcorners(1,:);

%Create node matrices, first layer is north value for that coordinate,
%second is east
nodes = zeros(cells_vert,cells_horiz,2);
for i=1:cells_vert
    for j=1:cells_horiz
        nodes(i,j,1) = (i-1)*(top_edge(j,1)-bottom_edge(j,1))/(cells_vert-1)+bottom_edge(j,1);
        nodes(i,j,2) = (i-1)*(top_edge(j,2)-bottom_edge(j,2))/(cells_vert-1)+bottom_edge(j,2);
    end
end

%Find closest grid point to vessel pose
[clist,rlist] = min(abs(nodes(:,:,1)-X)+abs(nodes(:,:,2)-Y));
[~,col] = min(clist);
row = rlist(col);
relPose = [row col];

%Find closest grid point to exit gate
exitPoint = (exitGate*2-1)*[(NEDcorners(4,1)-NEDcorners(3,1))/7 (NEDcorners(4,2)-NEDcorners(3,2))/7]+...
    NEDcorners(3,:);
[clist,rlist] = min(abs(nodes(:,:,1)-exitPoint(1))+abs(nodes(:,:,2)-exitPoint(2)));
[~,col] = min(clist);
row = rlist(col);
targetPt = [row col];

%% Populate obstacle grid

%Initialize obstacle grid size
obGrid = zeros(cells_vert,cells_horiz);

%Convert landmarks to NED coordinates
% NEDlandmarks = [(X+landmarks(:,1).*cos((Psi+landmarks(:,2))*pi/180)) (Y+landmarks(:,1).*sin((Psi+landmarks(:,2))*pi/180))];
%Find limits on north and east coordinates to remove landmarks from map
%that are from different tasks
Nmax = max(NEDcorners(:,1));
Nmin = min(NEDcorners(:,1));
Emax = max(NEDcorners(:,2));
Emin = min(NEDcorners(:,2));
%Mark landmarks out of bounded region
Nvalid = (NEDlandmarks(:,1)<Nmax & NEDlandmarks(:,1)>Nmin);
Evalid = (NEDlandmarks(:,2)<Emax & NEDlandmarks(:,2)>Emin);
NEbounded = Nvalid & Evalid;
NEDlandmarks(~NEbounded,:) = NaN;

%Relative coordinates for padding
neighbors_rel = [1,-1;1,0;1,1;0,1;-1,1;-1,0;-1,-1;0,-1];
%Find closest location for each of the landmarks in the obstacle grid
valid_landmark_idx = find(~isnan(NEDlandmarks(:,1)));
for q = 1:length(valid_landmark_idx)
    k = valid_landmark_idx(q);
    [clist,rlist] = min(abs(nodes(:,:,1)-NEDlandmarks(k,1))+abs(nodes(:,:,2)-NEDlandmarks(k,2)));
    [~,col] = min(clist);
    row = rlist(col);
    %Mark as obstacle
    obGrid(row,col) = -1;
    %Find grid coordinates for padding
    neighbors_abs = neighbors_rel + ones(8,1)*[row col];
    %Mark invalid indices
    neighbors_invalidX = (neighbors_abs(:,1)<=0) | (neighbors_abs(:,1)>cells_vert);
    neighbors_invalidY = (neighbors_abs(:,2)<=0) | (neighbors_abs(:,2)>cells_horiz);
    neighbors_invalid = neighbors_invalidX | neighbors_invalidY;
    neighbors_abs(neighbors_invalid,:) = NaN;
    %Track neighbors that are obstacles
    neighbors_obstacles = (obGrid(neighbors_abs(~neighbors_invalid,1)+...
        cells_vert*(neighbors_abs(~neighbors_invalid,2)-1)) == -1);
    neighbors_abs(neighbors_obstacles,:) = NaN;
    n_valid = ~isnan(neighbors_abs(:,1));
    %Flag padded area in obstacle grid, if already flagged, increase flag
    %val
    obGrid(neighbors_abs(n_valid,1)+cells_vert*(neighbors_abs(n_valid,2)-1)) = 2+...
        obGrid(neighbors_abs(n_valid,1)+cells_vert*(neighbors_abs(n_valid,2)-1));
end

end

== matlab function RobotX_SLAMdataCollect/Main FSM/Path/Path To Trajectory ==
  data: time input; valid output; relPose input; trajectory output; Path input; nodes input
function [valid, trajectory] = PathToTrajectory(time, relPose, Path, nodes)
%Written By Anderson Lebbad on September 8, 2014

%This code takes the output path from the A*, the node map, and the
%relative pose of the vessel, and outputs a trajectory for the low level
%controller.

%% Initialize output
valid = 0;
trajectory = zeros(8,2);

%Time tracking variable for updating valid flag
persistent lastTime
if isempty(lastTime)
    lastTime = time - 5;
end

%% Determine grid points

num_on_path = sum(~isnan(Path(:,1)));
if num_on_path > 1
    
    %Find the closest location in the path to the current point
    [~,closestIdx] = min(abs(Path(:,1)-relPose(1))+abs(Path(:,2)-relPose(2)));
    
    %Find how many points there are past the initial in the path
    num_remaining = num_on_path - closestIdx + 1;
    
    %Find the last path point to pass
    if num_remaining > 8
        initIdx = closestIdx + 1;
        lastIdx = initIdx + 7;
        
        %Grab points
        points = Path(initIdx:lastIdx,:);
        
        %% Convert to NED and output
        
        %Find the NED coordinates of those grid points, and write output
        [m,n] = size(nodes(:,:,1));
        trajectory(:,1) = nodes(points(:,1)+m*(points(:,2)-1));
        trajectory(:,2) = nodes(points(:,1)+m*(points(:,2)-1)+m*n);
        %Check timing to flag valid
        timeDiff = time - lastTime;
        if timeDiff >= 5
            valid = 1;
            lastTime = time;
        end
    end
end

end
